simulink model "unstAirfoilAero_sim_example_drag"  (R2018b)
settings: Solver=FixedStepAuto  StartTime=0.0  StopTime=t_sim  FixedStep=0.002  RelTol=1e-3
values from neighbouring files (symbols this model uses):
  a = V./Ma    [unstAirfoilAero.m]    (also in unstAirfoilAeroFast.m; unstAirfoilAero_example_drag.m = 300)
  airfoil = airfoilAnalyticSimpleCreate('airfoilAnalyticSimple_params_default')    [unstAirfoilAero_example_drag.m]
  alpha_0 = 0    [unstAirfoilAero_example_drag.m]
  c = 1    [unstAirfoilAero_example.m]    (also in unstAirfoilAero_example_drag.m = 2.8)
  Delta_alpha = 8    [unstAirfoilAero_example_drag.m]
  k = logspace( -4,log10(0.3),100 )    [unstAirfoilAero_example.m]    (also in unstAirfoilAero_example_drag.m = 0.0378)
  V = 1    [unstAirfoilAero_example.m]    (also in unstAirfoilAero_example_drag.m = 120)
settings Model: Creator=Ybeyer  LastModifiedBy=yannic

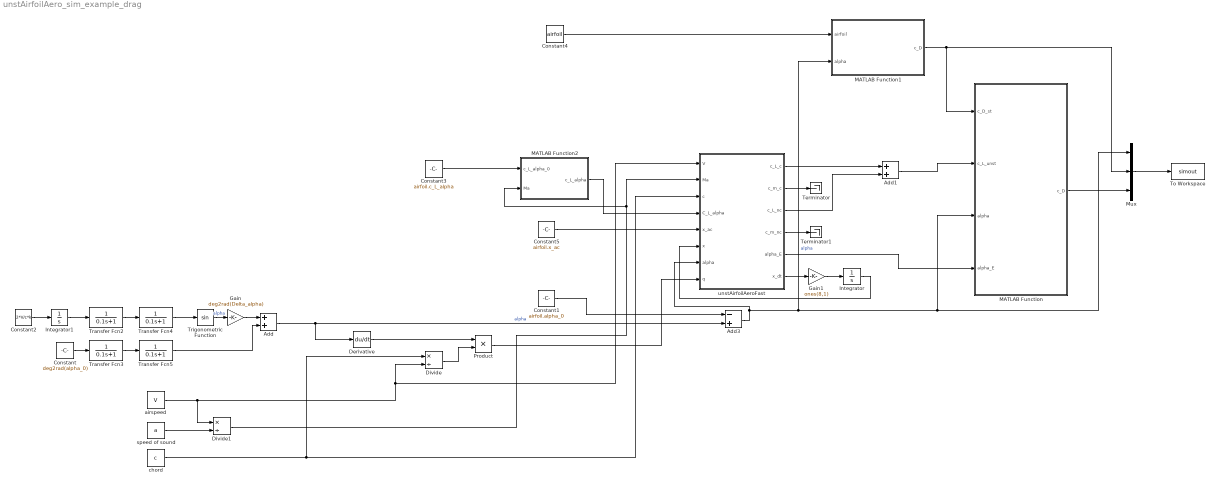
== system unstAirfoilAero_sim_example_drag ==
  Add : Sum
  Add1 : Sum
  Add3 : Sum  Inputs=-+
  Constant : Constant  Value=deg2rad(alpha_0)
  Constant1 : Constant  Value=airfoil.alpha_0
  Constant2 : Constant  Value=2*V/c*k
  Constant3 : Constant  Value=airfoil.c_L_alpha
  Constant4 : Constant  Value=airfoil  OutDataTypeStr=Bus: airfoil_bus
  Constant5 : Constant  Value=airfoil.x_ac
  Derivative : Derivative
  Divide : Product  Inputs=*/
  Divide1 : Product  Inputs=*/
  Gain : Gain  Gain=deg2rad(Delta_alpha)
  Gain1 : Gain  Gain=ones(8,1)
  Integrator : Integrator
  Integrator1 : Integrator
  MATLAB Function : MATLAB Function  TreatAsAtomicUnit=on
  MATLAB Function1 : MATLAB Function  TreatAsAtomicUnit=on
  MATLAB Function2 : MATLAB Function  TreatAsAtomicUnit=on
  Mux : Mux  Inputs=3
  Product : Product
  Terminator : Terminator
  Terminator1 : Terminator
  To Workspace : ToWorkspace  VariableName=simout  SaveFormat=Timeseries  SampleTime=-1
  Transfer Fcn{2..5} (4 alike) : TransferFcn  Denominator=[0.1 1]
  Trigonometric Function : Trigonometry
  airspeed : Constant  Value=V
  chord : Constant  Value=c
  speed of sound : Constant  Value=a
  unstAirfoilAeroFast : MATLAB Function  TreatAsAtomicUnit=on
  wires:
  chord/1 -> unstAirfoilAeroFast/3(c), Divide/1
  Divide/1 -> Product/2
  Product/1 -> unstAirfoilAeroFast/8(q)
  speed of sound/1 -> Divide1/2
  Derivative/1 -> Product/1
  Add/1 -> Add3/2, Derivative/1  "alpha"
  Trigonometric Function/1 -> Gain/1  "alpha"
  Constant/1 -> Transfer Fcn3/1
  Gain/1 -> Add/1
  Transfer Fcn3/1 -> Transfer Fcn5/1
  Transfer Fcn2/1 -> Transfer Fcn4/1
  Integrator1/1 -> Transfer Fcn2/1
  Constant2/1 -> Integrator1/1
  Transfer Fcn4/1 -> Trigonometric Function/1
  Transfer Fcn5/1 -> Add/2
  Add3/1 -> MATLAB Function/3(alpha), Mux/1, MATLAB Function1/2(alpha), unstAirfoilAeroFast/7(alpha)  "alpha"
  unstAirfoilAeroFast/4(c_m_nc) -> Terminator1/1
  unstAirfoilAeroFast/3(c_L_nc) -> Add1/2
  unstAirfoilAeroFast/2(c_m_c) -> Terminator/1
  unstAirfoilAeroFast/1(c_L_c) -> Add1/1
  airspeed/1 -> Divide/2, unstAirfoilAeroFast/1(V), Divide1/1
  Integrator/1 -> unstAirfoilAeroFast/6(x)
  Constant5/1 -> unstAirfoilAeroFast/5(x_ac)
  Constant1/1 -> Add3/1
  MATLAB Function2/1(c_L_alpha) -> unstAirfoilAeroFast/4(C_L_alpha)
  unstAirfoilAeroFast/6(x_dt) -> Gain1/1
  unstAirfoilAeroFast/5(alpha_E) -> MATLAB Function/4(alpha_E)
  Divide1/1 -> unstAirfoilAeroFast/2(Ma), MATLAB Function2/2(Ma)
  MATLAB Function1/1(c_D) -> MATLAB Function/1(c_D_st), Mux/2
  Constant4/1 -> MATLAB Function1/1(airfoil)
  Gain1/1 -> Integrator/1
  MATLAB Function/1(c_D) -> Mux/3
  Mux/1 -> To Workspace/1
  Constant3/1 -> MATLAB Function2/1(c_L_alpha_0)
  Add1/1 -> MATLAB Function/2(c_L_unst)

== matlab function unstAirfoilAero_sim_example_drag/MATLAB Function1 ==
  data: airfoil input; c_D output; alpha input
function c_D = airfoilAnalyticSimpleCd( airfoil, alpha )
c_D = airfoilAnalyticSimpleCd( airfoil, alpha );
end

== matlab function unstAirfoilAero_sim_example_drag/MATLAB Function ==
  data: c_D_st input; c_L_unst input; alpha input; c_D output; alpha_E input
function c_D = unstAirfoilAeroCd( c_D_st, c_L_unst, alpha, alpha_E )
c_D = unstAirfoilAeroCd( c_D_st, c_L_unst, alpha, alpha_E );
end

== matlab function unstAirfoilAero_sim_example_drag/MATLAB Function2 ==
  data: c_L_alpha_0 input; c_L_alpha output; Ma input
function c_L_alpha = fcn(c_L_alpha_0,Ma)

c_L_alpha = c_L_alpha_0 * 1/sqrt(1-Ma^2);

end

== matlab function unstAirfoilAero_sim_example_drag/unstAirfoilAeroFast ==
  data: V input; c_L_c output; Ma input; c input; C_L_alpha input; x_ac input; c_m_c output; c_L_nc output; c_m_nc output; x input; alpha input; q input; alpha_E output; x_dt output
function [c_L_c,c_m_c,c_L_nc,c_m_nc,alpha_E,x_dt] = unstAirfoilAeroFast( ...
    V, Ma, c, C_L_alpha, x_ac, x, alpha, q ) %#codegen
[c_L_c,c_m_c,c_L_nc,c_m_nc,alpha_E,x_dt] = unstAirfoilAeroFast( ...
    V, Ma, c, C_L_alpha, x_ac, x, alpha, q );
end
